simulink model "HighTemperatureOven_Simulink2019b"  (R2020b)
settings: Solver=ode4  StartTime=0.0  StopTime=SIM_TIME  FixedStep=STEP_SIZE  RelTol=1e-3
undefined symbols (not defined in the file): Cg, Cs, k, kc, kg, kr, Tg0K, Ts0K, umax, umin
settings Model: Creator=Mikkel  LastModifiedBy=roga
settings DataIOCC: LimitDataPoints=on  SaveFormat=Array  ReturnWorkspaceOutputs=off
settings OptimizationCC: ExpressionDepthLimit=2147483647  LifeSpan=inf
settings DebuggingCC: UnderspecifiedInitializationDetection=Classic  MergeDetectMultiDrivingBlocksExec=none  SolverPrmCheckMsg=warning  FcnCallInpInsideContextMsg=warning  StateNameClashWarn=warning  SFUnexpectedBacktrackingDiag=warning  SFNoUnconditionalDefaultTransitionDiag=warning  SFExecutionAtInitializationDiag=none  ArithmeticOperatorsInVariantConditions=warning
settings HardwareCC: ProdBitPerPointer=32  ProdBitPerSizeT=32  ProdBitPerPtrDiffT=32  ProdLargestAtomicFloat=None  ProdIntDivRoundTo=Undefined  ProdEndianess=Unspecified  ProdWordSize=32  ProdHWDeviceType=32-bit Generic
settings ModelReferenceCC: PropagateSignalLabelsOutOfModel=off
settings SFSimCC: SimUseLocalCustomCode=off  CustomCodeUndefinedFunction=UseInterfaceOnly
settings RTWCC: RTWUseLocalCustomCode=off
settings CodeAppCC: StateflowObjectComments=on
settings GRTTargetCC: TargetLangStandard=C89/C90 (ANSI)  CombineOutputUpdateFcns=off  GRTInterface=on
settings ConfigComp: CovMetricSettings=dw  CovSaveCumulativeToWorkspaceVar=on  CovSaveSingleToWorkspaceVar=on  CovExternalEMLEnable=off  CovSFcnEnable=off

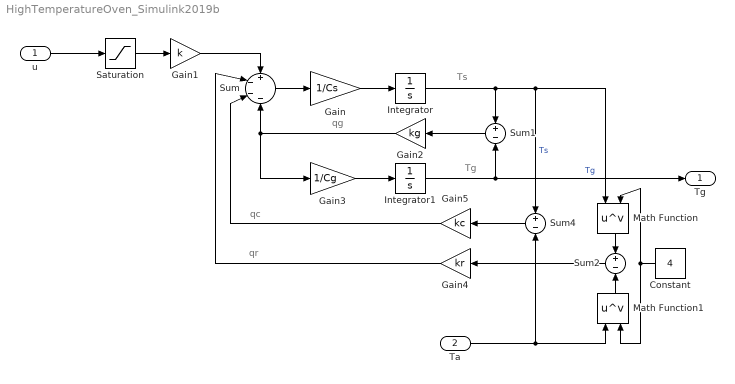
== system HighTemperatureOven_Simulink2019b ==
  note: qg
  note: Ts
  note: Tg
  note: qr
  note: qc
  u : Inport
  Ta : Inport  Port=2
  Constant : Constant  Value=4
  Gain : Gain  Gain=1/Cs
  Gain1 : Gain  Gain=k
  Gain2 : Gain  Gain=kg
  Gain3 : Gain  Gain=1/Cg
  Gain4 : Gain  Gain=kr
  Gain5 : Gain  Gain=kc
  Integrator : Integrator  Priority=1  InitialCondition=Ts0K
  Integrator1 : Integrator  Priority=2  InitialCondition=Tg0K
  Math Function : Math  Operator=pow  SignedPower=on  SaturateOnIntegerOverflow=on
  Math Function1 : Math  Operator=pow  SignedPower=on  SaturateOnIntegerOverflow=on
  Saturation : Saturate  UpperLimit=umax  LowerLimit=umin
  Sum : Sum  Inputs=+---
  Sum1 : Sum  Inputs=+-
  Sum2 : Sum  Inputs=+-
  Sum4 : Sum  Inputs=+-
  Tg : Outport
  wires:
  Gain/1 -> Integrator/1
  Sum/1 -> Gain/1
  Integrator/1 -> Sum1/1, Sum4/1, Math Function/1  "Ts"
  Sum1/1 -> Gain2/1
  Gain2/1 -> Gain3/1, Sum/4
  Gain3/1 -> Integrator1/1
  Integrator1/1 -> Sum1/2, Tg/1  "Tg"
  Gain4/1 -> Sum/2
  Sum2/1 -> Gain4/1
  Gain1/1 -> Sum/1
  Math Function/1 -> Sum2/1
  Constant/1 -> Math Function/2, Math Function1/2
  Math Function1/1 -> Sum2/2
  Sum4/1 -> Gain5/1
  Gain5/1 -> Sum/3
  Ta/1 -> Math Function1/1, Sum4/2
  Saturation/1 -> Gain1/1
  u/1 -> Saturation/1
